simulink model "Copy_of_Rocket_test"  (R2019b)
settings: Solver=VariableStepAuto  StartTime=0.0  StopTime=10  RelTol=1e-3
InitFcn:
  | initScript
undefined symbols (not defined in the file): aeng, Anoz, C_IE0, C_LE, Omega_earth, P, r0, Thrust, v0, x0
settings Model: Creator=frizzer  LastModifiedBy=frizzer

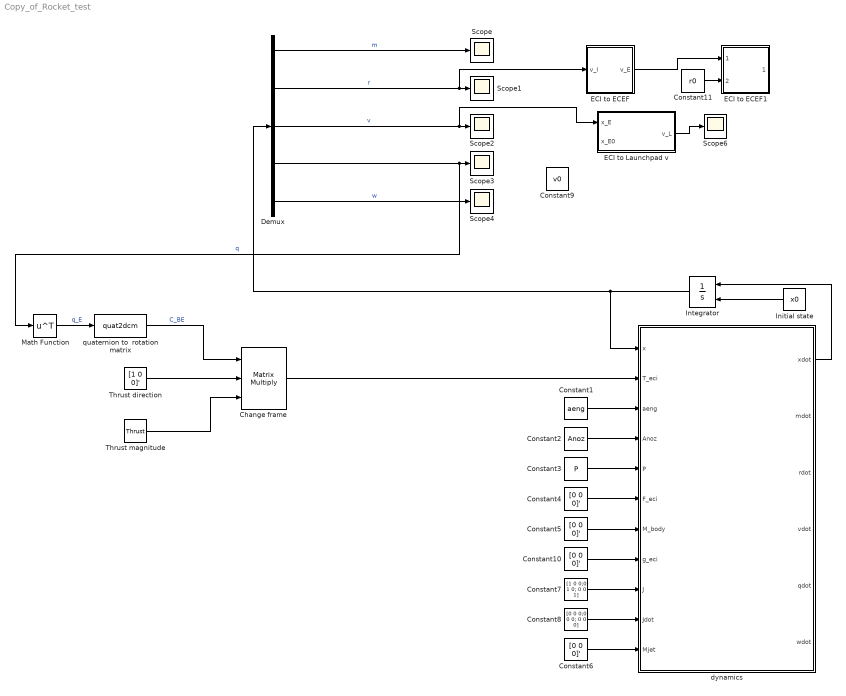
== system Copy_of_Rocket_test ==
  Change frame : Product  Inputs=3  Multiplication=Matrix(*)
  Constant1 : Constant  Value=aeng
  Constant{4..6,10} (4 alike) : Constant  Value=[0 0 0]'
  Constant11 : Constant  Value=r0
  Constant2 : Constant  Value=Anoz
  Constant3 : Constant  Value=P
  Constant7 : Constant  Value=[1 0 0;0 1 0; 0 0 1]
  Constant8 : Constant  Value=[0 0 0;0 0 0; 0 0 0]
  Constant9 : Constant  Value=v0
  Demux : Demux  Outputs=[1 3 3 4 3]
  ECI to ECEF : Subsystem
  ECI to ECEF1 : Subsystem
  ECI to Launchpad v : Subsystem
  Initial state : Constant  Value=x0
  Integrator : Integrator  InitialConditionSource=external  InitialCondition=x0
  Math Function : Math  Operator=transpose  SignedPower=off  SaturateOnIntegerOverflow=on
  Scope{,1..4,6} (6 alike) : Scope
  Thrust direction : Constant  Value=[1 0 0]'
  Thrust magnitude : Constant  Value=Thrust
  dynamics : MATLAB Function  TreatAsAtomicUnit=on
  quaternion to  rotation matrix : MATLABFcn  MATLABFcn=quat2dcm  Output1D=off
  wires:
  Thrust magnitude/1 -> Change frame/3
  Thrust direction/1 -> Change frame/2
  Change frame/1 -> dynamics/2(T_eci)
  Integrator/1 -> Demux/1, dynamics/1(x)
  Initial state/1 -> Integrator/2
  Constant1/1 -> dynamics/3(aeng)
  Constant2/1 -> dynamics/4(Anoz)
  Constant3/1 -> dynamics/5(P)
  dynamics/1(xdot) -> Integrator/1
  Demux/1 -> Scope/1  "m"
  Demux/2 -> ECI to ECEF/1("v_I "), Scope1/1  "r"
  Demux/3 -> ECI to Launchpad v/1(x_E), Scope2/1  "v"
  Demux/4 -> Scope3/1, Math Function/1  "q"
  Demux/5 -> Scope4/1  "w"
  Constant4/1 -> dynamics/6(F_eci)
  Constant5/1 -> dynamics/7(M_body)
  Constant7/1 -> dynamics/9(J)
  Constant8/1 -> dynamics/10(Jdot)
  Constant6/1 -> dynamics/11(Mjet)
  Constant10/1 -> dynamics/8(g_eci)
  Math Function/1 -> quaternion to  rotation matrix/1  "q_E"
  quaternion to  rotation matrix/1 -> Change frame/1  "C_BE"
  ECI to Launchpad v/1(v_L) -> Scope6/1
  ECI to ECEF/1(v_E) -> ECI to ECEF1/1("vector_E ")
  Constant11/1 -> ECI to ECEF1/2("origin_E ")

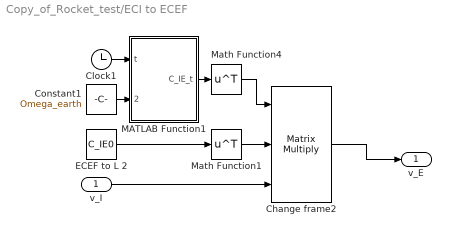
== system Copy_of_Rocket_test/ECI to ECEF ==
  "v_I " : Inport
  Change frame2 : Product  Inputs=3  Multiplication=Matrix(*)
  Clock1 : Clock
  Constant1 : Constant  Value=Omega_earth
  ECEF to L 2 : Constant  Value=C_IE0
  MATLAB Function1 : MATLAB Function  TreatAsAtomicUnit=on
  Math Function1 : Math  Operator=transpose  SignedPower=off  SaturateOnIntegerOverflow=on
  Math Function4 : Math  Operator=transpose  SignedPower=off  SaturateOnIntegerOverflow=on
  v_E : Outport
  wires:
  Math Function4/1 -> Change frame2/1
  "v_I "/1 -> Change frame2/3
  Constant1/1 -> MATLAB Function1/2(Omega_earth)
  MATLAB Function1/1(C_IE_t) -> Math Function4/1
  Clock1/1 -> MATLAB Function1/1(t)
  Change frame2/1 -> v_E/1
  ECEF to L 2/1 -> Math Function1/1
  Math Function1/1 -> Change frame2/2

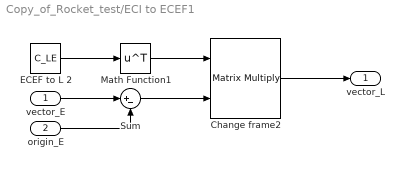
== system Copy_of_Rocket_test/ECI to ECEF1 ==
  "vector_E " : Inport
  "origin_E " : Inport  Port=2
  Change frame2 : Product  Multiplication=Matrix(*)
  ECEF to L 2 : Constant  Value=C_LE
  Math Function1 : Math  Operator=transpose  SignedPower=off  SaturateOnIntegerOverflow=on
  Sum : Sum  Inputs=|+-
  vector_L : Outport
  wires:
  ECEF to L 2/1 -> Math Function1/1
  Change frame2/1 -> vector_L/1
  "vector_E "/1 -> Sum/1
  Math Function1/1 -> Change frame2/1
  Sum/1 -> Change frame2/2
  "origin_E "/1 -> Sum/2

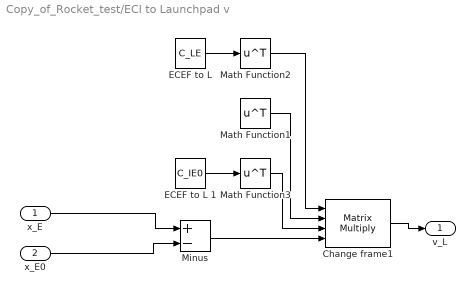
== system Copy_of_Rocket_test/ECI to Launchpad v ==
  x_E : Inport
  x_E0 : Inport  Port=2
  Change frame1 : Product  Inputs=4  Multiplication=Matrix(*)
  "ECEF to L " : Constant  Value=C_LE
  ECEF to L 1 : Constant  Value=C_IE0
  Math Function1 : Math  Operator=transpose  SignedPower=off  SaturateOnIntegerOverflow=on
  Math Function2 : Math  Operator=transpose  SignedPower=off  SaturateOnIntegerOverflow=on
  Math Function3 : Math  Operator=transpose  SignedPower=off  SaturateOnIntegerOverflow=on
  Minus : Sum  Inputs=+-
  v_L : Outport
  wires:
  Math Function1/1 -> Change frame1/2
  ? -> Math Function1/1
  Change frame1/1 -> v_L/1
  x_E/1 -> Minus/1
  "ECEF to L "/1 -> Math Function2/1
  Math Function2/1 -> Change frame1/1
  Minus/1 -> Change frame1/4
  x_E0/1 -> Minus/2
  ECEF to L 1/1 -> Math Function3/1
  Math Function3/1 -> Change frame1/3

== matlab function Copy_of_Rocket_test/dynamics ==
  data: x input; xdot output; T_eci input; aeng input; Anoz input; P input; F_eci input; M_body input; g_eci input; J input; Jdot input; Mjet input; mdot output; rdot output; vdot output; qdot output; wdot output
function [xdot, mdot, rdot, vdot, qdot, wdot] = dynamics(x,T_eci,aeng,Anoz,P,F_eci,M_body,g_eci,J,Jdot,Mjet)

% INPUTS
% x      - state vector
% T_eci  - thrust force in ECI frame
% aeng   - mass depletion constant (Isp*g0)^-1
% Anoz   - engine nozzle area
% P      - atmospheric pressure
% F_eci  - sum of non-propulsive forces in ECI frame
% M_body - sum of moments in body frame
% g_eci  - gravity acceleration in ECI frame
% J      - inertia matrix
% Jdot   - inertia matrix derivative
% Mjet   - engine jet damping moment

% State vector
m=x(1);
r=x(2:4);
v=x(5:7);
q=x(8:11);
w=x(12:14);

% Propulsion
T=norm(T_eci);
mdot=-aeng*(T+P*Anoz);

% Translational ECI
F=T_eci+F_eci+m*g_eci;
vdot=F/m;
rdot=v;

% Quaternions
qdot=1/2*[q(4) -q(3)  q(2);
          q(3)  q(4) -q(1);
         -q(2)  q(1)  q(4);
         -q(1) -q(2) -q(3)]*w;

% Rotational BODY
M=M_body-Mjet-Jdot*w;
wdot=J\(-sksim(w)*J*w+M);

% State derivative -> to be integrated
xdot=[mdot;rdot;vdot;qdot;wdot];

end


function M=sksim(w)

M=[   0 -w(3) w(2);
    w(3)   0 -w(1);
   -w(2) w(1)   0];

end

== matlab function Copy_of_Rocket_test/ECI to ECEF/MATLAB Function1 ==
  data: t input; C_IE_t output; Omega_earth input
function C_IE_t=ECI2ECEF(t,Omega_earth)
   C_IE_t =  [cos(Omega_earth*t)     sin(Omega_earth*t)  0;...
             -sin(Omega_earth*t)    cos(Omega_earth*t)  0;...
             0                      0                   1];
end
